simulink model "Simulation_Model"  (R2023a)
settings: Solver=daessc  StartTime=0.0  StopTime=5  RelTol=1e-3
undefined symbols (not defined in the file): t_sample
libraries: Code_Gen_lib x1, SignalEditorBlockLib x1, Simulation_lib x1
settings Model: SimulationMode=accelerator  Creator=FIRSTMentor  LastModifiedBy=FIRSTMentor
settings DebuggingCC: UnderspecifiedInitializationDetection=Classic  MergeDetectMultiDrivingBlocksExec=none
settings ModelReferenceCC: PropagateSignalLabelsOutOfModel=off

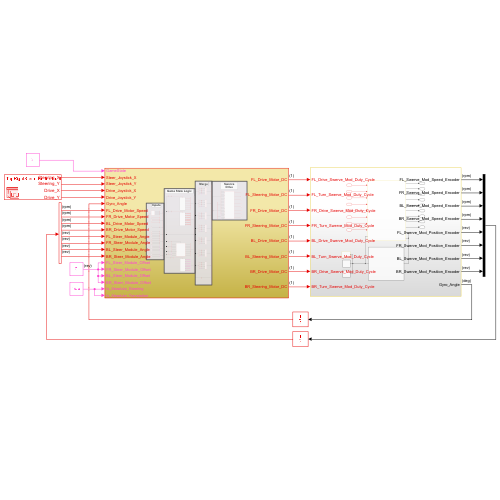
[thumbnail: Simulink's stored preview of the top-level diagram]
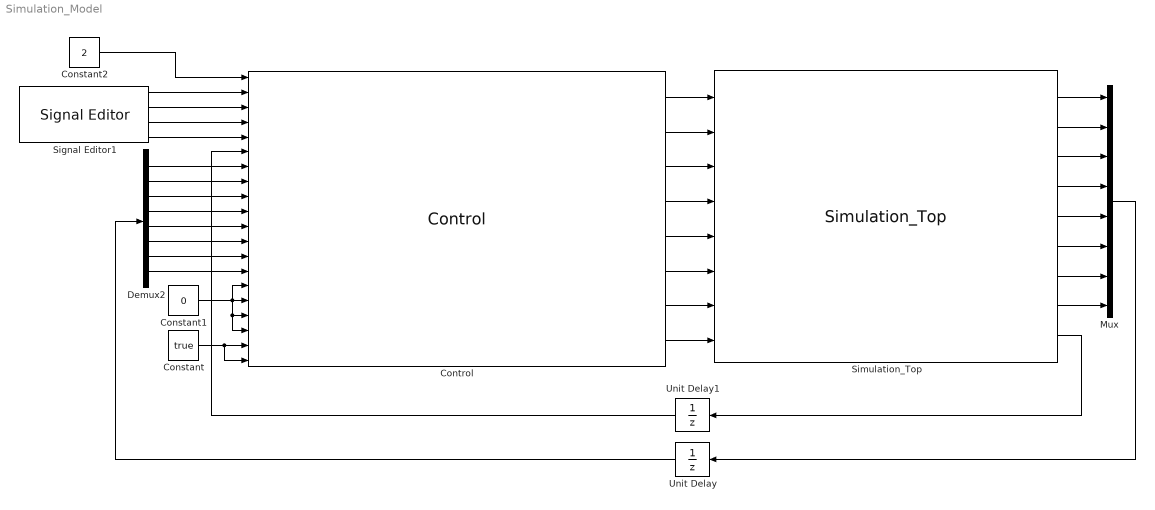
== system Simulation_Model ==
  Constant : Constant  Value=true
  Constant1 : Constant  Value=0
  Constant2 : Constant  Value=2
  Control : Code_Gen_lib/Control  SystemSampleTime=-1  VariantActivationTime=update diagram  Latency=0  AutoFrameSizeCalculation=off
  Demux2 : Demux  Outputs=8
  Mux : Mux  Inputs=8
  Signal Editor1 : SignalEditorBlockLib/Signal Editor  FileName=Joystick_input_test_data.mat  ActiveScenario=TopRightSteer_BottomLeftDrive  ActiveSignal=Steering_Y  IsBus=off  OutputBusObjectStr=Bus: BusObject  SampleTime=t_sample  Interpolate=off  ZeroCross=off  OutputAfterFinalValue=Setting to zero  Unit=inherit  PreserveSignalName=on  ApplySigPropsToAllScenarios=on
  Simulation_Top : Simulation_lib/Simulation_Top  SystemSampleTime=-1  VariantActivationTime=update diagram  Latency=0  AutoFrameSizeCalculation=off
  Unit Delay : UnitDelay  InitialCondition=[0 0 0 0 0 0 0 0]  SampleTime=t_sample  HasFrameUpgradeWarning=on
  Unit Delay1 : UnitDelay  SampleTime=t_sample  HasFrameUpgradeWarning=on
  wires:
  Control/3 -> Simulation_Top/3
  Control/2 -> Simulation_Top/2
  Control/4 -> Simulation_Top/4
  Control/1 -> Simulation_Top/1
  Control/5 -> Simulation_Top/5
  Control/6 -> Simulation_Top/6
  Control/7 -> Simulation_Top/7
  Control/8 -> Simulation_Top/8
  Simulation_Top/5 -> Mux/5
  Simulation_Top/4 -> Mux/4
  Simulation_Top/6 -> Mux/6
  Simulation_Top/3 -> Mux/3
  Simulation_Top/7 -> Mux/7
  Simulation_Top/2 -> Mux/2
  Simulation_Top/8 -> Mux/8
  Simulation_Top/1 -> Mux/1
  Demux2/1 -> Control/7
  Demux2/2 -> Control/8
  Demux2/3 -> Control/9
  Demux2/4 -> Control/10
  Demux2/5 -> Control/11
  Demux2/6 -> Control/12
  Demux2/7 -> Control/13
  Demux2/8 -> Control/14
  Mux/1 -> Unit Delay/1
  Unit Delay/1 -> Demux2/1
  Constant/1 -> Control/20, Control/19
  Simulation_Top/9 -> Unit Delay1/1
  Unit Delay1/1 -> Control/6
  Constant1/1 -> Control/15, Control/17, Control/18, Control/16
  Constant2/1 -> Control/1
  Signal Editor1/1 -> Control/2
  Signal Editor1/2 -> Control/3
  Signal Editor1/3 -> Control/4
  Signal Editor1/4 -> Control/5
